simulink model "TorqueReductionSignal"  (Simulink 8.2)
settings: Solver=ode45  StartTime=0.0  StopTime=10.0  RelTol=1e-3
model workspace (MAT data in the model file):
  demand_reduction_req = Simulink.Parameter
  demand_reduction_req.Value = 0.2
  demand_reduction_req.DataType = 'double'
settings Model: Creator=meta  LastModifiedBy=tiwari
settings DataIOCC: SignalLoggingSaveFormat=Dataset
settings OptimizationCC: ExpressionDepthLimit=128
settings DebuggingCC: FcnCallInpInsideContextMsg=EnableAllAsError
settings GRTTargetCC: CombineOutputUpdateFcns=on  GRTInterface=off

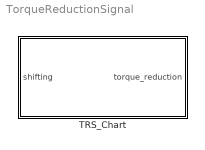
== system TorqueReductionSignal ==
  TRS_Chart : Subsystem

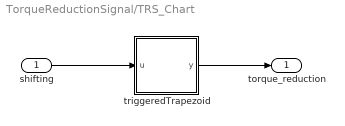
== system TorqueReductionSignal/TRS_Chart ==
  shifting : Inport  OutDataTypeStr=boolean
  triggeredTrapezoid : Stateflow chart  TreatAsAtomicUnit=on
  torque_reduction : Outport  OutDataTypeStr=double
  wires:
  shifting/1 -> triggeredTrapezoid/1(u)
  triggeredTrapezoid/1(y) -> torque_reduction/1

== stateflow chart TRS_Chart/triggeredTrapezoid ==
  settings: description=|
      | <?xml version="1.0" encoding="utf-8"?>
      | <ltlProperties AbsenceCount="3" ResponseCount="2">
      |    <ltlProperty afterExpr="" beforeExpr="" expr="[](!((y &lt; -0.2) || (y &gt; 1)))" id="Absence1" name="AbsenceProperty" rawProperty="(y &lt; -0.2) || (y &gt; 1)" rawProperty2="" scope="Global" type="Absence"/>
      |    <ltlProperty afterExpr="" beforeExpr="" expr="[](!((y &lt; 0) || (y &gt; 1)))" id="Absence2" name="AbsenceProperty1" rawProperty="(y &lt; 0) || (y &gt; 1)" rawProperty2="" scope="Global" type="Absence"/>
      |    <ltlProperty afterExpr="" beforeExpr="" expr="[](!((y &lt; 0.9) || (y &gt; 1)))" id="Absence3" name="AbsenceProperty12" rawProperty="(y &lt; 0.9) || (y &gt; 1)" rawProperty2="" scope="Global" type="Absence"/>
      |    <ltlProperty afterExpr="" beforeExpr="" expr="[]((G(shifting)) -&gt; &lt;&gt;(y = 0.8))" id="Response1" name="ResponseProperty" rawProperty="G(shifting)" rawProperty2="y = 0.8" scope="Global" type="Response"/>
      |    <ltlProperty afterExpr="" beforeExpr="" expr="[]((G(!(shifting))) -&gt; &lt;&gt;(y = 1))" id="Response2" name="ResponseProperty4" rawProperty="G(!(shifting))" rawProperty2="y = 1" scope="Global" type="Response"/>
      | </ltlProperties>
  state Low
    entry: y = offset;
  state Rising
    during: y = y + rise_step;
  state Falling
    during: y = y - fall_step;
  state High
    entry: y = amplitude+offset;
  (default) -> Low : / rise_step = amplitude / (rise_time / sample_period);
      |  fall_step = amplitude / (fall_time / sample_period);
  Falling -> Low [order 1] : [y <= offset]
  Low -> Rising : [u == true]
  Rising -> Falling [order 2] : [u==false]
  Rising -> High [order 1] : [y >= amplitude+offset]
  Falling -> Rising [order 2] : [u==true]
  High -> Falling : [u == false]
  data: sample_period local double =0.01; u input boolean; amplitude local double =-0.2; rise_time local double =0.01; fall_time local double =0.05; offset local double =1; rise_step local double =0.0; fall_step local double =0.0; y output double =0
